simulink model "two_level_spwm"  (R2016a)
settings: Solver=VariableStepAuto  StartTime=0.0  StopTime=stop_time  RelTol=1e-3
values from neighbouring files (symbols this model uses):
  DCLINK_Cap1 = 100e-6    (= 0.0001)    [spectrumanalysis.m]
  Lload = Xload/ref_frequency    [spectrumanalysis.m]
  ma = 0.9    [spectrumanalysis.m]
  ref_frequency = 2*pi*50    (= 314.159265359)    [spectrumanalysis.m]
  Rload = Zload*Load_Power_Factor    [spectrumanalysis.m]
  Sampling_time = 1/(20*sw_frequency)    (= 2.43902439024e-05)    [spectrumanalysis.m]
  Vin = DC_Voltage_Source + Rin*(Load_Real_Power/DC_Voltage_Source)    (= 555.740740741)    [spectrumanalysis.m]
libraries: powerlib x22, simulink x6, powerlib_meascontrol x5
settings Model: Creator=hakan  LastModifiedBy=hakan
settings DataIOCC: LimitDataPoints=on
settings DebuggingCC: MaxConsecutiveZCsMsg=none  AllowSymbolicDim=off
settings ModelReferenceCC: PropagateSignalLabelsOutOfModel=off
settings GRTTargetCC: GeneratePreprocessorConditionals=Use local settings

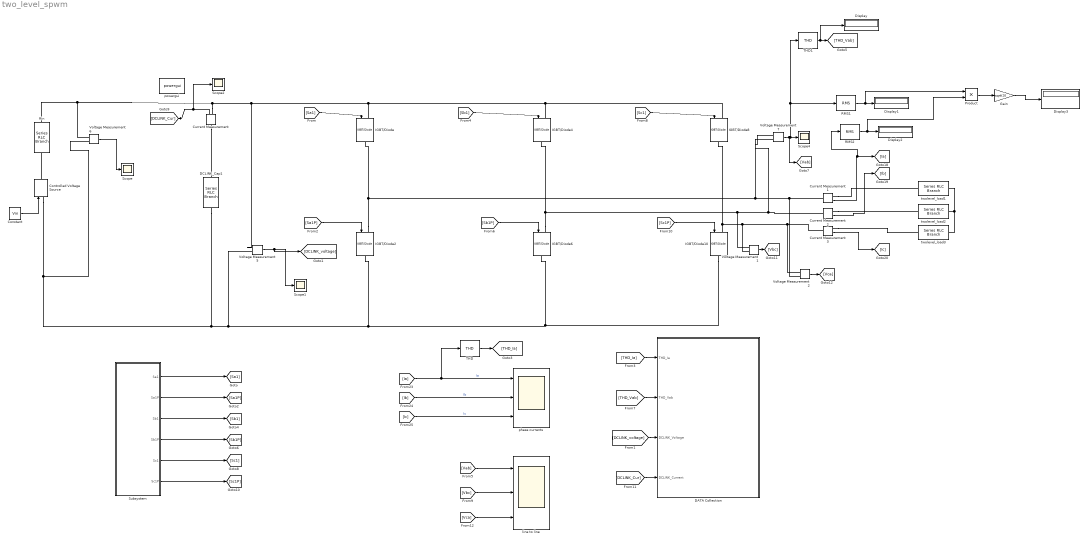
== system two_level_spwm ==
  Constant : Constant  Value=Vin
  Controlled Voltage Source : powerlib/Electrical Sources/Controlled Voltage Source  Initialize=on  Source_Type=AC  Amplitude=0  Phase=0  Frequency=0  Measurements=None
  Current Measurement{,1..3} (4 alike) : powerlib/Measurements/Current Measurement  PhasorSimulation=off  OutputType=Complex  PSBequivalent=0
  DATA Collection : Subsystem
  DCLINK_Cap1 : powerlib/Elements/Series RLC Branch  LConnTagsString=__new0  RConnTagsString=__new0  BranchType=C  Resistance=1  Inductance=1e-3  SetiL0=off  InitialCurrent=0  Capacitance=DCLINK_Cap1  Setx0=off  InitialVoltage=0  Measurements=None
  Display{,1..3} (4 alike) : Display
  Gain : Gain  Gain=sqrt(3)
  IGBT/Diode{,2,4,6,8,10} (6 alike) : powerlib/Power Electronics/IGBT//Diode  Ron=1e-3  Rs=1e5  Cs=inf  Measurements=off
  Product : Product
  RMS1 : powerlib_meascontrol/Measurements/RMS  TrueRMS=off  Freq=50  RMSInit=120  Ts=0
  RMS2 : powerlib_meascontrol/Measurements/RMS  TrueRMS=off  Freq=50  RMSInit=120  Ts=0
  Rin : powerlib/Elements/Series RLC Branch  LConnTagsString=__new0  RConnTagsString=__new0  BranchType=R  Resistance=1  Inductance=1e-3  SetiL0=off  InitialCurrent=0  Capacitance=1000e-6  Setx0=off  InitialVoltage=0  Measurements=None
  Scope{,1..2,4} (4 alike) : Scope
  Subsystem : Subsystem
  THD : powerlib_meascontrol/Measurements/THD  Freq=50  Ts=0
  THD1 : powerlib_meascontrol/Measurements/THD  Freq=50  Ts=0
  Voltage Measurement{1..2,5..7} (5 alike) : powerlib/Measurements/Voltage Measurement  PhasorSimulation=off  OutputType=Complex  PSBequivalent=0
  line to line : Scope  NumInputPorts=3
  phase currents : Scope  NumInputPorts=3
  powergui : powerlib/powergui  Priority=1  SimulationMode=Discrete  SolverType=Tustin  SampleTime=Sampling_time  frequency=60  SPID=off  DisableSnubberDevices=off  DisableRonSwitches=off  DisableVfSwitches=off  SwTol=0  DisplayEquations=off  Interpol=off  ExternalGateDelay=off  methode=off  Ts=10  FunctionMessages=off  echomessages=off  HookPort=off  EnableUseOfTLC=off  x0status=blocks  frequencyindice=0  Pbase=100e6  ErrMax=1e-4  Iterations=50  UnitsV=kV  UnitsW=MW  buscounter=0  RestoreLinks=warning  ResistiveCurrentMeasurement=off  Frange=[0:2:500]  Ylog=off  Xlog=on  ShowGrid=off  save=off  variable=ZData  structure=Phase_currents  ZoomFFT=off  StartTime=0.1  cycles=5  DisplayStyle=1  fundamental=50  FreqAxis=off  MaxFrequency=2000  frequencyindicesteady=1  RmsSteady=1  display=off
  twolevel_load1 : powerlib/Elements/Series RLC Branch  LConnTagsString=__new0  RConnTagsString=__new0  BranchType=RL  Resistance=Rload  Inductance=Lload  SetiL0=off  InitialCurrent=0  Capacitance=1e-6  Setx0=off  InitialVoltage=0  Measurements=None
  twolevel_load2 : powerlib/Elements/Series RLC Branch  LConnTagsString=__new0  RConnTagsString=__new0  BranchType=RL  Resistance=Rload  Inductance=Lload  SetiL0=off  InitialCurrent=0  Capacitance=1e-6  Setx0=off  InitialVoltage=0  Measurements=None
  twolevel_load3 : powerlib/Elements/Series RLC Branch  LConnTagsString=__new0  RConnTagsString=__new0  BranchType=RL  Resistance=Rload  Inductance=Lload  SetiL0=off  InitialCurrent=0  Capacitance=1e-6  Setx0=off  InitialVoltage=0  Measurements=None
  wires:
  Subsystem/1("Sa1 ") -> [Sa1]
  Subsystem/2(Sa1P) -> [Sa1P]
  Subsystem/3(Sb1) -> [Sb1]
  Subsystem/6(Sc1P) -> [Sc1P]
  Subsystem/5(Sc1) -> [Sc1]
  Subsystem/4(Sb1P) -> [Sb1P]
  [Sa1] -> IGBT/Diode/1
  [Sa1P] -> IGBT/Diode2/1
  [Sb1] -> IGBT/Diode4/1
  [Sb1P] -> IGBT/Diode6/1
  [Sc1] -> IGBT/Diode8/1
  [Sc1P] -> IGBT/Diode10/1
  Current Measurement1/1 -> RMS2/1, [Ia]
  Current Measurement2/1 -> [Ib]
  Current Measurement3/1 -> [Ic]
  [Ib] -> phase currents/2  "Ib"
  [Ia] -> phase currents/1, THD/1  "Ia"
  [Ic] -> phase currents/3  "Ic"
  Voltage Measurement5/1 -> Scope1/1, [DCLINK_voltage]
  THD/1 -> [THD_Ia]
  [THD_Ia] -> DATA Collection/1(THD_Ia)
  [THD_Vab] -> DATA Collection/2(THD_Vab)
  [DCLINK_voltage] -> DATA Collection/3(DCLINK_Voltage)
  Current Measurement/1 -> Scope2/1, [DCLINK_Cur]
  [DCLINK_Cur] -> DATA Collection/4(DCLINK_Current)
  RMS1/1 -> Product/1, Display1/1
  RMS2/1 -> Product/2, Display2/1
  Product/1 -> Gain/1
  Gain/1 -> Display3/1
  Voltage Measurement7/1 -> [Vab], THD1/1, RMS1/1, Scope4/1
  Constant/1 -> Controlled Voltage Source/1
  Voltage Measurement6/1 -> Scope/1
  THD1/1 -> Display/1, [THD_Vab]
  Voltage Measurement1/1 -> [Vbc]
  Voltage Measurement2/1 -> [Vca]
  [Vab] -> line to line/1
  [Vca] -> line to line/3
  [Vbc] -> line to line/2
  connections:
  Current Measurement/RConn1 -- Voltage Measurement6/LConn1 -- Rin/LConn1 -- Voltage Measurement5/LConn1 -- IGBT/Diode4/LConn1 -- IGBT/Diode8/LConn1 -- IGBT/Diode/LConn1
  Voltage Measurement5/LConn2 -- IGBT/Diode2/RConn1 -- IGBT/Diode10/RConn1 -- IGBT/Diode6/RConn1 -- Voltage Measurement6/LConn2 -- Controlled Voltage Source/LConn1 -- DCLINK_Cap1/RConn1
  IGBT/Diode2/LConn1 -- Voltage Measurement2/LConn2 -- Current Measurement1/LConn1 -- Voltage Measurement7/LConn1 -- IGBT/Diode/RConn1
  IGBT/Diode6/LConn1 -- Voltage Measurement7/LConn2 -- Current Measurement2/LConn1 -- Voltage Measurement1/LConn1 -- IGBT/Diode4/RConn1
  IGBT/Diode8/RConn1 -- Voltage Measurement2/LConn1 -- Current Measurement3/LConn1 -- Voltage Measurement1/LConn2 -- IGBT/Diode10/LConn1
  Current Measurement1/RConn1 -- twolevel_load1/LConn1
  Current Measurement3/RConn1 -- twolevel_load3/LConn1
  Current Measurement2/RConn1 -- twolevel_load2/LConn1
  Current Measurement/LConn1 -- DCLINK_Cap1/LConn1
  twolevel_load1/RConn1 -- twolevel_load3/RConn1 -- twolevel_load2/RConn1
  Controlled Voltage Source/RConn1 -- Rin/RConn1

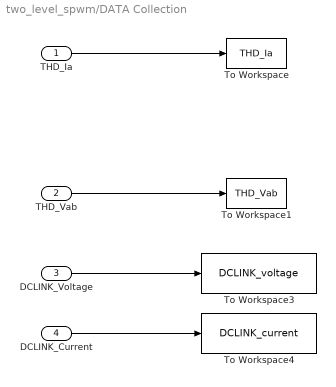
== system two_level_spwm/DATA Collection ==
  THD_Ia : Inport
  THD_Vab : Inport  Port=2
  DCLINK_Voltage : Inport  Port=3
  DCLINK_Current : Inport  Port=4
  To Workspace : ToWorkspace  VariableName=THD_Ia  SaveFormat=Timeseries  SampleTime=-1
  To Workspace1 : ToWorkspace  VariableName=THD_Vab  SaveFormat=Timeseries  SampleTime=-1
  To Workspace3 : ToWorkspace  VariableName=DCLINK_voltage  SaveFormat=Timeseries  SampleTime=-1
  To Workspace4 : ToWorkspace  VariableName=DCLINK_current  SaveFormat=Timeseries  SampleTime=-1
  wires:
  DCLINK_Voltage/1 -> To Workspace3/1
  THD_Ia/1 -> To Workspace/1
  THD_Vab/1 -> To Workspace1/1
  DCLINK_Current/1 -> To Workspace4/1

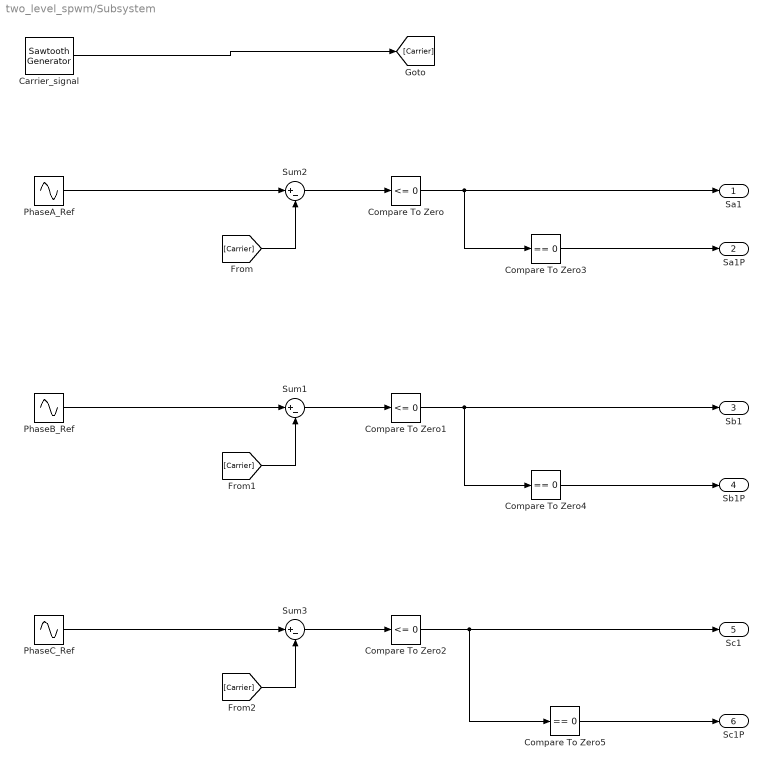
== system two_level_spwm/Subsystem ==
  Carrier_signal : powerlib_meascontrol/Pulse & Signal Generators/Sawtooth Generator  Freq=sw_frequency  Phase=180  Ts=0
  Compare To Zero : simulink/Logic and Bit Operations/Compare To Zero  relop=<=  OutDataTypeStr=boolean  ZeroCross=off
  Compare To Zero1 : simulink/Logic and Bit Operations/Compare To Zero  relop=<=  OutDataTypeStr=boolean  ZeroCross=off
  Compare To Zero2 : simulink/Logic and Bit Operations/Compare To Zero  relop=<=  OutDataTypeStr=boolean  ZeroCross=off
  Compare To Zero3 : simulink/Logic and Bit Operations/Compare To Zero  relop===  OutDataTypeStr=boolean  ZeroCross=off
  Compare To Zero4 : simulink/Logic and Bit Operations/Compare To Zero  relop===  OutDataTypeStr=boolean  ZeroCross=off
  Compare To Zero5 : simulink/Logic and Bit Operations/Compare To Zero  relop===  OutDataTypeStr=boolean  ZeroCross=off
  PhaseA_Ref : Sin  Amplitude=ma  Frequency=ref_frequency  SampleTime=0
  PhaseB_Ref : Sin  Amplitude=ma  Frequency=ref_frequency  Phase=-2*pi/3  SampleTime=0
  PhaseC_Ref : Sin  Amplitude=ma  Frequency=ref_frequency  Phase=2*pi/3  SampleTime=0
  Sum1 : Sum  Inputs=|+-
  Sum2 : Sum  Inputs=|+-
  Sum3 : Sum  Inputs=|+-
  "Sa1 " : Outport
  Sa1P : Outport  Port=2
  Sb1 : Outport  Port=3
  Sb1P : Outport  Port=4
  Sc1 : Outport  Port=5
  Sc1P : Outport  Port=6
  wires:
  PhaseA_Ref/1 -> Sum2/1
  Compare To Zero/1 -> Compare To Zero3/1, "Sa1 "/1
  Sum2/1 -> Compare To Zero/1
  [Carrier] -> Sum2/2
  Compare To Zero1/1 -> Compare To Zero4/1, Sb1/1
  PhaseB_Ref/1 -> Sum1/1
  [Carrier] -> Sum1/2
  Compare To Zero2/1 -> Compare To Zero5/1, Sc1/1
  PhaseC_Ref/1 -> Sum3/1
  [Carrier] -> Sum3/2
  Sum1/1 -> Compare To Zero1/1
  Sum3/1 -> Compare To Zero2/1
  Compare To Zero3/1 -> Sa1P/1
  Compare To Zero4/1 -> Sb1P/1
  Compare To Zero5/1 -> Sc1P/1
  Carrier_signal/1 -> [Carrier]
